simulink model "FCW_Harness"  (R2022b)
settings: Solver=VariableStepAuto  StartTime=0.0  StopTime=10.0  RelTol=1e-3
undefined symbols (not defined in the file or in its folder): tc_distance, tc_expectedRed, tc_expectedSafe, tc_expectedYellow, tc_targetInLane, tc_targetPresent, tc_vrel
settings Model: Creator=HP  LastModifiedBy=HP

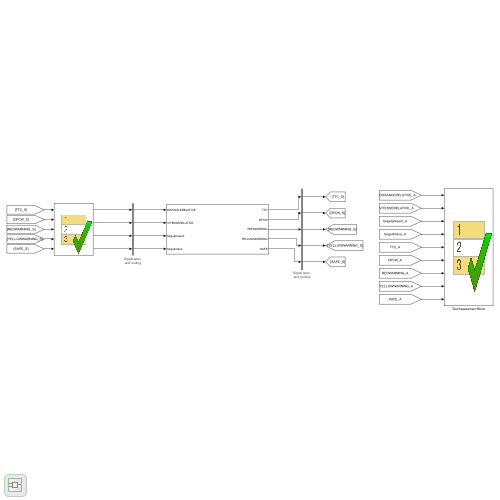
[thumbnail: Simulink's stored preview of the top-level diagram]
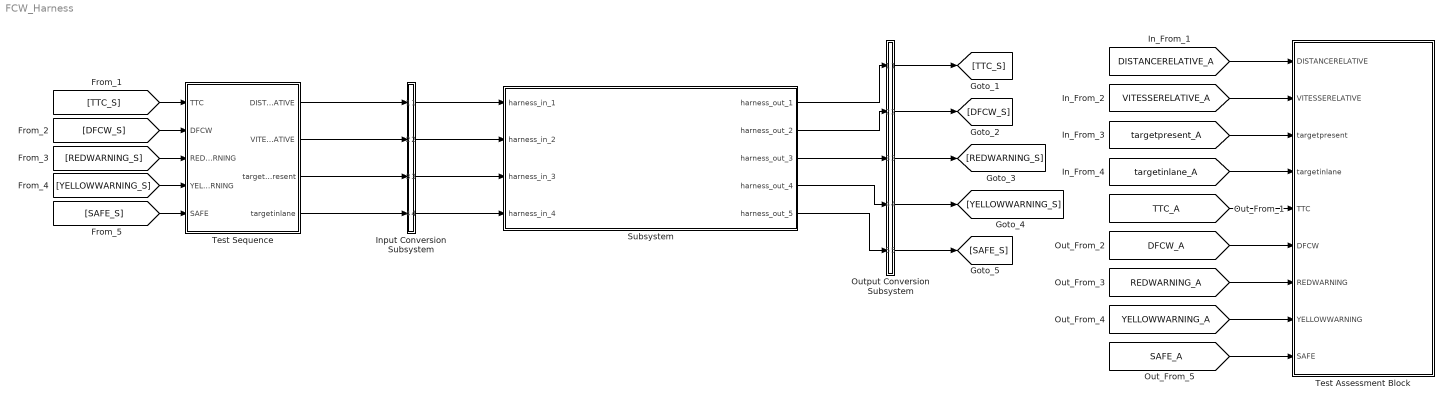
== system FCW_Harness ==
  Input Conversion Subsystem : Subsystem  Tag=__SLT_ICS__  Description=|
      | Signal spec.
      | and routing
      settings: AttributesFormatString=%<Description>
  Output Conversion Subsystem : Subsystem  Tag=__SLT_OCS__  Description=|
      | Signal spec.
      | and routing
      settings: AttributesFormatString=%<Description>
  Subsystem : Subsystem  Tag=__SL_testing_harness_stub_
  Test Assessment Block : Test Sequence  Tag=__SLT_ASMT__  TreatAsAtomicUnit=on
  Test Sequence : Test Sequence  TreatAsAtomicUnit=on
  wires:
  [DISTANCERELATIVE_A] -> Test Assessment Block/1(DISTANCERELATIVE)
  [VITESSERELATIVE_A] -> Test Assessment Block/2(VITESSERELATIVE)
  [targetpresent_A] -> Test Assessment Block/3(targetpresent)
  [targetinlane_A] -> Test Assessment Block/4(targetinlane)
  [TTC_A] -> Test Assessment Block/5(TTC)
  [DFCW_A] -> Test Assessment Block/6(DFCW)
  [REDWARNING_A] -> Test Assessment Block/7(REDWARNING)
  [YELLOWWARNING_A] -> Test Assessment Block/8(YELLOWWARNING)
  [SAFE_A] -> Test Assessment Block/9(SAFE)
  Test Sequence/1(DISTANCERELATIVE) -> Input Conversion Subsystem/1(Inport_1)
  Test Sequence/2(VITESSERELATIVE) -> Input Conversion Subsystem/2(Inport_2)
  Test Sequence/3(targetpresent) -> Input Conversion Subsystem/3(Inport_3)
  Test Sequence/4(targetinlane) -> Input Conversion Subsystem/4(Inport_4)
  [TTC_S] -> Test Sequence/1(TTC)
  [DFCW_S] -> Test Sequence/2(DFCW)
  [REDWARNING_S] -> Test Sequence/3(REDWARNING)
  [YELLOWWARNING_S] -> Test Sequence/4(YELLOWWARNING)
  [SAFE_S] -> Test Sequence/5(SAFE)
  Output Conversion Subsystem/1(Outport_1) -> [TTC_S]
  Output Conversion Subsystem/2(Outport_2) -> [DFCW_S]
  Output Conversion Subsystem/3(Outport_3) -> [REDWARNING_S]
  Output Conversion Subsystem/4(Outport_4) -> [YELLOWWARNING_S]
  Output Conversion Subsystem/5(Outport_5) -> [SAFE_S]
  Input Conversion Subsystem/1(Outport_1) -> Subsystem/1(harness_in_1)
  Input Conversion Subsystem/2(Outport_2) -> Subsystem/2(harness_in_2)
  Input Conversion Subsystem/3(Outport_3) -> Subsystem/3(harness_in_3)
  Input Conversion Subsystem/4(Outport_4) -> Subsystem/4(harness_in_4)
  Subsystem/1(harness_out_1) -> Output Conversion Subsystem/1(Inport_1)
  Subsystem/2(harness_out_2) -> Output Conversion Subsystem/2(Inport_2)
  Subsystem/3(harness_out_3) -> Output Conversion Subsystem/3(Inport_3)
  Subsystem/4(harness_out_4) -> Output Conversion Subsystem/4(Inport_4)
  Subsystem/5(harness_out_5) -> Output Conversion Subsystem/5(Inport_5)

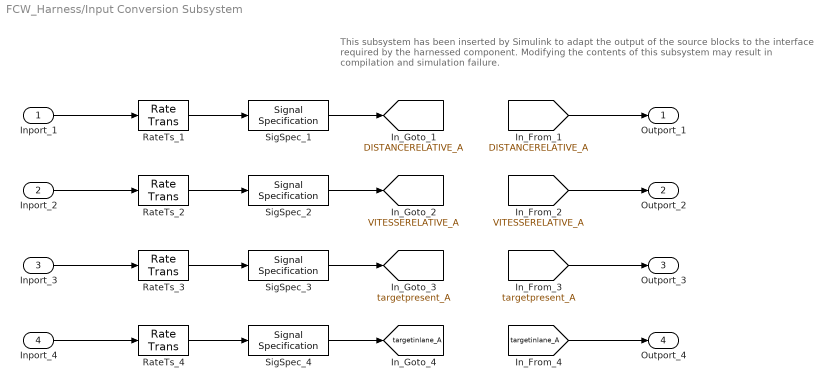
== system FCW_Harness/Input Conversion Subsystem ==
  note: This subsystem has been inserted by Simulink to adapt the output of the source blocks to the interface required by the harnessed component.
      |  Modifying the contents of this subsystem may result in compilation and simulation failure.
  Inport_1 : Inport
  Inport_2 : Inport  Port=2
  Inport_3 : Inport  Port=3
  Inport_4 : Inport  Port=4
  RateTs_{1..4} (4 alike) : RateTransition  OutPortSampleTime=[-1, 0]
  SigSpec_{1..4} (4 alike) : SignalSpecification  OutDataTypeStr=double  Dimensions=[1]  SampleTime=[-1, 0]
  Outport_1 : Outport
  Outport_2 : Outport  Port=2
  Outport_3 : Outport  Port=3
  Outport_4 : Outport  Port=4
  tag scope: DISTANCERELATIVE_A=global, VITESSERELATIVE_A=global, targetinlane_A=global, targetpresent_A=global
  wires:
  [DISTANCERELATIVE_A] -> Outport_1/1
  SigSpec_1/1 -> [DISTANCERELATIVE_A]
  RateTs_1/1 -> SigSpec_1/1
  Inport_1/1 -> RateTs_1/1
  [VITESSERELATIVE_A] -> Outport_2/1
  SigSpec_2/1 -> [VITESSERELATIVE_A]
  RateTs_2/1 -> SigSpec_2/1
  Inport_2/1 -> RateTs_2/1
  [targetpresent_A] -> Outport_3/1
  SigSpec_3/1 -> [targetpresent_A]
  RateTs_3/1 -> SigSpec_3/1
  Inport_3/1 -> RateTs_3/1
  [targetinlane_A] -> Outport_4/1
  SigSpec_4/1 -> [targetinlane_A]
  RateTs_4/1 -> SigSpec_4/1
  Inport_4/1 -> RateTs_4/1

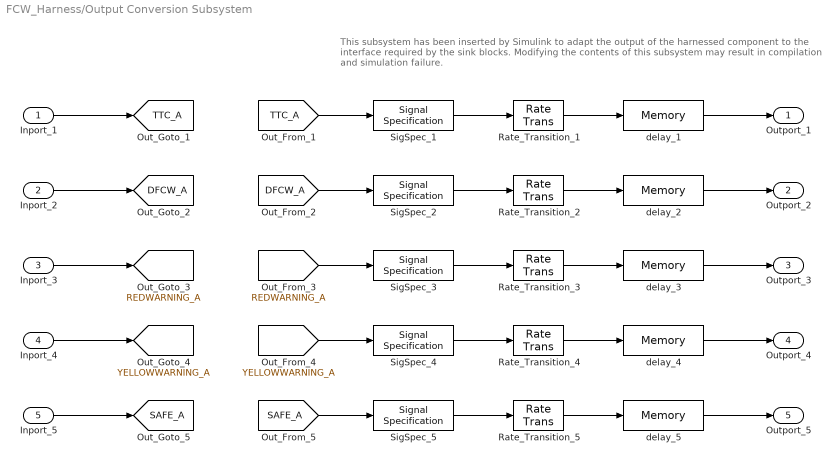
== system FCW_Harness/Output Conversion Subsystem ==
  note: This subsystem has been inserted by Simulink to adapt the output of the harnessed component to the interface required by the sink blocks.
      |  Modifying the contents of this subsystem may result in compilation and simulation failure.
  Inport_1 : Inport
  Inport_2 : Inport  Port=2
  Inport_3 : Inport  Port=3
  Inport_4 : Inport  Port=4
  Inport_5 : Inport  Port=5
  Rate_Transition_{1..5} (5 alike) : RateTransition  OutPortSampleTimeOpt=Inherit
  SigSpec_1 : SignalSpecification  OutDataTypeStr=double  Dimensions=[1]
  SigSpec_2 : SignalSpecification  OutDataTypeStr=double  Dimensions=[1]
  SigSpec_3 : SignalSpecification  OutDataTypeStr=boolean  Dimensions=[1, 1]
  SigSpec_4 : SignalSpecification  OutDataTypeStr=boolean  Dimensions=[1, 1]
  SigSpec_5 : SignalSpecification  OutDataTypeStr=boolean  Dimensions=[1, 1]
  delay_{1..5} (5 alike) : Memory
  Outport_1 : Outport
  Outport_2 : Outport  Port=2
  Outport_3 : Outport  Port=3
  Outport_4 : Outport  Port=4
  Outport_5 : Outport  Port=5
  tag scope: DFCW_A=global, REDWARNING_A=global, SAFE_A=global, TTC_A=global, YELLOWWARNING_A=global
  wires:
  Inport_1/1 -> [TTC_A]
  [TTC_A] -> SigSpec_1/1
  SigSpec_1/1 -> Rate_Transition_1/1
  Rate_Transition_1/1 -> delay_1/1
  delay_1/1 -> Outport_1/1
  Inport_2/1 -> [DFCW_A]
  [DFCW_A] -> SigSpec_2/1
  SigSpec_2/1 -> Rate_Transition_2/1
  Rate_Transition_2/1 -> delay_2/1
  delay_2/1 -> Outport_2/1
  Inport_3/1 -> [REDWARNING_A]
  [REDWARNING_A] -> SigSpec_3/1
  SigSpec_3/1 -> Rate_Transition_3/1
  Rate_Transition_3/1 -> delay_3/1
  delay_3/1 -> Outport_3/1
  Inport_4/1 -> [YELLOWWARNING_A]
  [YELLOWWARNING_A] -> SigSpec_4/1
  SigSpec_4/1 -> Rate_Transition_4/1
  Rate_Transition_4/1 -> delay_4/1
  delay_4/1 -> Outport_4/1
  Inport_5/1 -> [SAFE_A]
  [SAFE_A] -> SigSpec_5/1
  SigSpec_5/1 -> Rate_Transition_5/1
  Rate_Transition_5/1 -> delay_5/1
  delay_5/1 -> Outport_5/1

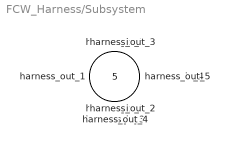
== system FCW_Harness/Subsystem ==
  harness_in_1 : Inport
  harness_in_2 : Inport  Port=2
  harness_in_3 : Inport  Port=3
  harness_in_4 : Inport  Port=4
  harness_out_1 : Outport
  harness_out_2 : Outport  Port=2
  harness_out_3 : Outport  Port=3
  harness_out_4 : Outport  Port=4
  harness_out_5 : Outport  Port=5

== stateflow chart FCW_Harness/Test Assessment Block ==
  state Run
    state step_1_1
    state step_1_2
      verify(SAFE == tc_expectedSafe);
      verify(REDWARNING == tc_expectedRed);
      verify(YELLOWWARNING == tc_expectedYellow);
    (default) -> (junction 22)
    Run -> (junction 22)
    (junction 22) -> (junction 23) [order 1] : [t < 0.1
        | ]
    (junction 23) -> step_1_1 [order 1] : [~in(Run.step_1_1)]
    (junction 22) -> (junction 31) [order 2]
    (junction 23) -> (junction 26) [order 2]
    (junction 31) -> (junction 32)
    (junction 32) -> step_1_2 [order 1] : [~in(Run.step_1_2)]
    (junction 32) -> (junction 35) [order 2]
  (default) -> Run
  data: DISTANCERELATIVE input double size=[1]; VITESSERELATIVE input double size=[1]; targetpresent input double size=[1]; targetinlane input double size=[1]; TTC input double size=[1]; DFCW input double size=[1]; REDWARNING input boolean size=[1, 1]; YELLOWWARNING input boolean size=[1, 1]; SAFE input boolean size=[1, 1]; tc_expectedSafe parameter; tc_expectedYellow parameter; tc_expectedRed parameter

== stateflow chart FCW_Harness/Test Sequence ==
  settings: updateMethod=DISCRETE  sampleTime=0.2
  state Run
    %% Initialize data outputs.
    %% Scenario SAFE
    DISTANCERELATIVE = tc_distance;
    VITESSERELATIVE = tc_vrel;
    targetpresent = tc_targetPresent;
    targetinlane = tc_targetInLane;
  (default) -> Run
  data: TTC input double size=[1]; DFCW input double size=[1]; REDWARNING input boolean size=[1, 1]; YELLOWWARNING input boolean size=[1, 1]; SAFE input boolean size=[1, 1]; DISTANCERELATIVE output double size=[1]; VITESSERELATIVE output double size=[1]; targetpresent output double size=[1]; targetinlane output double size=[1]; tc_distance parameter; tc_vrel parameter; tc_targetPresent parameter; tc_targetInLane parameter
